simulink model "ES101A_DiagcMgr"  (R2013b)
settings: Solver=ode45  StartTime=0.0  StopTime=0.44  RelTol=1e-3
values from neighbouring files (symbols this model uses):
  BrdgVltg = DataDict.IpSignal    [ES101A_DiagcMgr_DataDict.m]
  DEM_CLEAR_PENDING = DataDict.Constant    [ES101A_DiagcMgr_DataDict.m]
  DEM_DTC_GROUP_ALL_DTCS = DataDict.Constant    [ES101A_DiagcMgr_DataDict.m]
  DFTAGICNTR_CNT_U08 = DataDict.Constant    [ES101A_DiagcMgr_DataDict.m]
  DIAGCMGR_NTCINFOSTSTESTFAILD_CNT_U08 = DataDict.Constant    [ES101A_DiagcMgr_DataDict.m]
  DIAGCMGR_NTCINFOSTSTESTFAILDTHISIGNCYC_CNT_U08 = DataDict.Constant    [ES101A_DiagcMgr_DataDict.m]
  DIAGCMGR_NTCINFOSTSTESTNOTCMPLTHISIGNCYC_CNT_U08 = DataDict.Constant    [ES101A_DiagcMgr_DataDict.m]
  DiagcMgrFltResp = DataDict.Calibration    [ES101A_DiagcMgr_DataDict.m]
  DiagcMgrNtcFltAry = DataDict.NVM    [ES101A_DiagcMgr_DataDict.m]
  DIAGCSTSCTRLDSHTDWNFLTPRSNT_CNT_U16 = DataDict.Constant    [ES101A_DiagcMgr_DataDict.m]
  DIAGCSTSDFTHWAG_CNT_U16 = DataDict.Constant    [ES101A_DiagcMgr_DataDict.m]
  DIAGCSTSDFTHWAGSERLCOMEXPRTVAL_CNT_U16 = DataDict.Constant    [ES101A_DiagcMgr_DataDict.m]
  DIAGCSTSDFTVEHSPD_CNT_U16 = DataDict.Constant    [ES101A_DiagcMgr_DataDict.m]
  DIAGCSTSININVAL_CNT_U16 = DataDict.Constant    [ES101A_DiagcMgr_DataDict.m]
  DIAGCSTSIVTR1INACTV_CNT_U16 = DataDict.Constant    [ES101A_DiagcMgr_DataDict.m]
  DIAGCSTSIVTR2INACTV_CNT_U16 = DataDict.Constant    [ES101A_DiagcMgr_DataDict.m]
  DIAGCSTSLIMDTPRFMNC_CNT_U16 = DataDict.Constant    [ES101A_DiagcMgr_DataDict.m]
  DIAGCSTSRAMPTOZEROFLTPRSNT_CNT_U16 = DataDict.Constant    [ES101A_DiagcMgr_DataDict.m]
  DIAGCSTSWHLIMBREJCTNDI_CNT_U16 = DataDict.Constant    [ES101A_DiagcMgr_DataDict.m]
  DTCIDXSTSFAIL_CNT_U08 = DataDict.Constant    [ES101A_DiagcMgr_DataDict.m]
  DTCIDXSTSNONTC_CNT_U08 = DataDict.Constant    [ES101A_DiagcMgr_DataDict.m]
  DTCIDXSTSNORES_CNT_U08 = DataDict.Constant    [ES101A_DiagcMgr_DataDict.m]
  DTCIDXSTSPASS_CNT_U08 = DataDict.Constant    [ES101A_DiagcMgr_DataDict.m]
  DTCIDXSTSUPDCFMD_CNT_U08 = DataDict.Constant    [ES101A_DiagcMgr_DataDict.m]
  ELECGLBPRM_IVTRCNT_CNT_U08 = DataDict.ConfigParam    [ES101A_DiagcMgr_DataDict.m]
  FLTINJ_DIAGCMGR_DIAGCSTSIVTR1INACTV = DataDict.Constant    [ES101A_DiagcMgr_DataDict.m]
  FLTINJ_DIAGCMGR_DIAGCSTSIVTR2INACTV = DataDict.Constant    [ES101A_DiagcMgr_DataDict.m]
  HwTq = DataDict.IpSignal    [ES101A_DiagcMgr_DataDict.m]
  IgnCntr = DataDict.IpSignal    [ES101A_DiagcMgr_DataDict.m]
  MAXDEBCNTRVAL_CNT_S16 = DataDict.Constant    [ES101A_DiagcMgr_DataDict.m]
  MAXRAMPRATE_ULSPERSEC_F32 = DataDict.Constant    [ES101A_DiagcMgr_DataDict.m]
  MINDEBCNTRVAL_CNT_S16 = DataDict.Constant    [ES101A_DiagcMgr_DataDict.m]
  MINRAMPRATE_ULSPERSEC_F32 = DataDict.Constant    [ES101A_DiagcMgr_DataDict.m]
  SCAMOTTQCMDTOONE_ULS_F32 = DataDict.Constant    [ES101A_DiagcMgr_DataDict.m]
  SCAMOTTQCMDTOZERO_ULS_F32 = DataDict.Constant    [ES101A_DiagcMgr_DataDict.m]
  SysSt = DataDict.IpSignal    [ES101A_DiagcMgr_DataDict.m]
  VehSpd = DataDict.IpSignal    [ES101A_DiagcMgr_DataDict.m]
undefined symbols (not defined in the file or in its folder): ActvMotTqCmdSca, ActvRampRate, AgiCntr, Dem_DTCFormatType, Dem_DTCOriginType, Dem_EventStatusType, DiagcData, DiagcMgrNtcMap, DiagcSts, DtcEnaMask, EcuT, HistNtcFltAry, MicroDiagcData, MotTq, NtcNr, NtcNrWithResd1, NtcStInfo, ProxySetNtcData, Sts, SysSt1, TOTNROFDTC_CNT_U08
libraries: simulink x151, FloatToFixd x5, NxtrNvM x4
(part 13 of 13)

== system ES101A_DiagcMgr/DiagcMgr/SetNtcStsCore/NtcNr is Valid/Diagnostics Not Inhibited/NtcEnabled/NTCSTS_PREFAILD/Update NtcInfoSts, DebCntr and Process RampRate/DebCntr = MAXDEBCNTRVAL_CNT_S16/ProcessRampResponse and DiagcSts/RapidShutdown Fault/Atomic Section2/Update Scale2 ==
  Action Port : ActionPort
  CopyRight2 : Subsystem  Description=|  mask(Copyright Information){none=on}
      | Copyright info block.                                               
      |                                                                     
      | Place copyright information at the top of every subsystem in design.
      mask prompts: none "No parameters"
      mask help: Place copyright information at the top of every subsystem in design.
      mask Display:
      | NxtrConf = 'Nexteer Confidential';
      | 
      | sys = bdroot; %handle for the current model ("system")
      | first = get_param(sys,'Created');
      | first = first(end-3:end);  %year is last four digits
      | 
      | last = get_param(sys,'LastModifiedDate');
      | if isempty(last)
      |     last = datestr(now,'yyyy');
      | else
      |     last = last(end-3:end);
      | end
      | 
      | if strcmp(first,last)
      |     fprintf('%s -- Copyright %s Nexteer',NxtrConf,first)
      | else
      |     fprintf('%s -- %s%s- %s Nexteer',NxtrConf,char(169),first,last)
      | end
  Scale Motor Torque Command to Zero : Constant  Value=SCAMOTTQCMDTOZERO_ULS_F32  OutDataTypeStr=single
  DiagcMgrActvMotTqCmdSca : Outport
  wires:
  Scale Motor Torque Command to Zero/1 -> DiagcMgrActvMotTqCmdSca/1

== system ES101A_DiagcMgr/DiagcMgr/SetNtcStsCore/NtcNr is Valid/Diagnostics Not Inhibited/NtcEnabled/NTCSTS_PREFAILD/Update NtcInfoSts, DebCntr and Process RampRate/DebCntr = MAXDEBCNTRVAL_CNT_S16/ProcessRampResponse and DiagcSts/RapidShutdown Fault/Atomic Section2/Update Scale3 ==
  Action Port : ActionPort
  CopyRight2 : Subsystem  Description=|  mask(Copyright Information){none=on}
      | Copyright info block.                                               
      |                                                                     
      | Place copyright information at the top of every subsystem in design.
      mask prompts: none "No parameters"
      mask help: Place copyright information at the top of every subsystem in design.
      mask Display:
      | NxtrConf = 'Nexteer Confidential';
      | 
      | sys = bdroot; %handle for the current model ("system")
      | first = get_param(sys,'Created');
      | first = first(end-3:end);  %year is last four digits
      | 
      | last = get_param(sys,'LastModifiedDate');
      | if isempty(last)
      |     last = datestr(now,'yyyy');
      | else
      |     last = last(end-3:end);
      | end
      | 
      | if strcmp(first,last)
      |     fprintf('%s -- Copyright %s Nexteer',NxtrConf,first)
      | else
      |     fprintf('%s -- %s%s- %s Nexteer',NxtrConf,char(169),first,last)
      | end
  Scale Motor Torque Command to Zero : Constant  Value=SCAMOTTQCMDTOZERO_ULS_F32  OutDataTypeStr=single
  ProxySetNtcMotTqCmdSca : Outport
  wires:
  Scale Motor Torque Command to Zero/1 -> ProxySetNtcMotTqCmdSca/1

== system ES101A_DiagcMgr/DiagcMgr/SetNtcStsCore/NtcNr is Valid/Diagnostics Not Inhibited/NtcEnabled/NTCSTS_PREFAILD/Update NtcInfoSts, DebCntr and Process RampRate/DebCntr = MAXDEBCNTRVAL_CNT_S16/ProcessRampResponse and DiagcSts/TimedShutdown Fault/Atomic Section2/CopyRight2 ==

== system ES101A_DiagcMgr/DiagcMgr/SetNtcStsCore/NtcNr is Valid/Diagnostics Not Inhibited/NtcEnabled/NTCSTS_PREFAILD/Update NtcInfoSts, DebCntr and Process RampRate/DebCntr = MAXDEBCNTRVAL_CNT_S16/ProcessRampResponse and DiagcSts/TimedShutdown Fault/Atomic Section2/Update Ramp Rate ==
  RampRate : Inport
  Action Port : ActionPort
  CopyRight2 : Subsystem  Description=|  mask(Copyright Information){none=on}
      | Copyright info block.                                               
      |                                                                     
      | Place copyright information at the top of every subsystem in design.
      mask prompts: none "No parameters"
      mask help: Place copyright information at the top of every subsystem in design.
      mask Display:
      | NxtrConf = 'Nexteer Confidential';
      | 
      | sys = bdroot; %handle for the current model ("system")
      | first = get_param(sys,'Created');
      | first = first(end-3:end);  %year is last four digits
      | 
      | last = get_param(sys,'LastModifiedDate');
      | if isempty(last)
      |     last = datestr(now,'yyyy');
      | else
      |     last = last(end-3:end);
      | end
      | 
      | if strcmp(first,last)
      |     fprintf('%s -- Copyright %s Nexteer',NxtrConf,first)
      | else
      |     fprintf('%s -- %s%s- %s Nexteer',NxtrConf,char(169),first,last)
      | end
  DiagcMgrActvRampRate : Outport
  wires:
  RampRate/1 -> DiagcMgrActvRampRate/1

== system ES101A_DiagcMgr/DiagcMgr/SetNtcStsCore/NtcNr is Valid/Diagnostics Not Inhibited/NtcEnabled/NTCSTS_PREFAILD/Update NtcInfoSts, DebCntr and Process RampRate/DebCntr = MAXDEBCNTRVAL_CNT_S16/ProcessRampResponse and DiagcSts/TimedShutdown Fault/Atomic Section2/Update Ramp Rate1 ==
  RampRate : Inport
  Action Port : ActionPort
  CopyRight2 : Subsystem  Description=|  mask(Copyright Information){none=on}
      | Copyright info block.                                               
      |                                                                     
      | Place copyright information at the top of every subsystem in design.
      mask prompts: none "No parameters"
      mask help: Place copyright information at the top of every subsystem in design.
      mask Display:
      | NxtrConf = 'Nexteer Confidential';
      | 
      | sys = bdroot; %handle for the current model ("system")
      | first = get_param(sys,'Created');
      | first = first(end-3:end);  %year is last four digits
      | 
      | last = get_param(sys,'LastModifiedDate');
      | if isempty(last)
      |     last = datestr(now,'yyyy');
      | else
      |     last = last(end-3:end);
      | end
      | 
      | if strcmp(first,last)
      |     fprintf('%s -- Copyright %s Nexteer',NxtrConf,first)
      | else
      |     fprintf('%s -- %s%s- %s Nexteer',NxtrConf,char(169),first,last)
      | end
  ProxySetNtcActvRampRate : Outport
  wires:
  RampRate/1 -> ProxySetNtcActvRampRate/1

== system ES101A_DiagcMgr/DiagcMgr/SetNtcStsCore/NtcNr is Valid/Diagnostics Not Inhibited/NtcEnabled/NTCSTS_PREFAILD/Update NtcInfoSts, DebCntr and Process RampRate/DebCntr = MAXDEBCNTRVAL_CNT_S16/ProcessRampResponse and DiagcSts/TimedShutdown Fault/Atomic Section2/Update Scale2 ==
  Action Port : ActionPort
  CopyRight2 : Subsystem  Description=|  mask(Copyright Information){none=on}
      | Copyright info block.                                               
      |                                                                     
      | Place copyright information at the top of every subsystem in design.
      mask prompts: none "No parameters"
      mask help: Place copyright information at the top of every subsystem in design.
      mask Display:
      | NxtrConf = 'Nexteer Confidential';
      | 
      | sys = bdroot; %handle for the current model ("system")
      | first = get_param(sys,'Created');
      | first = first(end-3:end);  %year is last four digits
      | 
      | last = get_param(sys,'LastModifiedDate');
      | if isempty(last)
      |     last = datestr(now,'yyyy');
      | else
      |     last = last(end-3:end);
      | end
      | 
      | if strcmp(first,last)
      |     fprintf('%s -- Copyright %s Nexteer',NxtrConf,first)
      | else
      |     fprintf('%s -- %s%s- %s Nexteer',NxtrConf,char(169),first,last)
      | end
  Scale Motor Torque Command to Zero : Constant  Value=SCAMOTTQCMDTOZERO_ULS_F32  OutDataTypeStr=single
  DiagcMgrActvMotTqCmdSca : Outport
  wires:
  Scale Motor Torque Command to Zero/1 -> DiagcMgrActvMotTqCmdSca/1

== system ES101A_DiagcMgr/DiagcMgr/SetNtcStsCore/NtcNr is Valid/Diagnostics Not Inhibited/NtcEnabled/NTCSTS_PREFAILD/Update NtcInfoSts, DebCntr and Process RampRate/DebCntr = MAXDEBCNTRVAL_CNT_S16/ProcessRampResponse and DiagcSts/TimedShutdown Fault/Atomic Section2/Update Scale3 ==
  Action Port : ActionPort
  CopyRight2 : Subsystem  Description=|  mask(Copyright Information){none=on}
      | Copyright info block.                                               
      |                                                                     
      | Place copyright information at the top of every subsystem in design.
      mask prompts: none "No parameters"
      mask help: Place copyright information at the top of every subsystem in design.
      mask Display:
      | NxtrConf = 'Nexteer Confidential';
      | 
      | sys = bdroot; %handle for the current model ("system")
      | first = get_param(sys,'Created');
      | first = first(end-3:end);  %year is last four digits
      | 
      | last = get_param(sys,'LastModifiedDate');
      | if isempty(last)
      |     last = datestr(now,'yyyy');
      | else
      |     last = last(end-3:end);
      | end
      | 
      | if strcmp(first,last)
      |     fprintf('%s -- Copyright %s Nexteer',NxtrConf,first)
      | else
      |     fprintf('%s -- %s%s- %s Nexteer',NxtrConf,char(169),first,last)
      | end
  Scale Motor Torque Command to Zero : Constant  Value=SCAMOTTQCMDTOZERO_ULS_F32  OutDataTypeStr=single
  ProxySetNtcMotTqCmdSca : Outport
  wires:
  Scale Motor Torque Command to Zero/1 -> ProxySetNtcMotTqCmdSca/1

== system ES101A_DiagcMgr/DiagcMgr/DiagcMgrPer2/Normal Periodic Processing/For All DTCs/For Each DTC/Check If DTC Status has Changed/DTC Status Changed OR DTC Update NOT Confirmed/Update DTC Status/Dtc Status is Failed/Update 'DTC Index Update Confirmed' Bit/StdRtn is E_OK/Set Bit 7 (DTC Update Confirmed)/CopyRight2 ==

== system ES101A_DiagcMgr/DiagcMgr/DiagcMgrPer2/Normal Periodic Processing/For All DTCs/For Each DTC/Check If DTC Status has Changed/DTC Status Changed OR DTC Update NOT Confirmed/Update DTC Status/Dtc Status is Passed/Update 'DTC Index Update Confirmed' Bit/StdRtn is E_OK/Set Bit 7 (DTC Update Confirmed)/CopyRight2 ==

== system ES101A_DiagcMgr/DiagcMgr/SetNtcStsCore/NtcNr is Valid/Diagnostics Not Inhibited/NtcEnabled/NTCSTS_FAILD/Update ISO Bits, Parameter Byte and AgiCntr /Check to Update Snapshot Data/UpdSnpshtData/Snapshot Data Enabled/While /While NTC Matches or Run out of Index/CopyRight2 ==

== system ES101A_DiagcMgr/DiagcMgr/SetNtcStsCore/NtcNr is Valid/Diagnostics Not Inhibited/NtcEnabled/NTCSTS_FAILD/Update ISO Bits, Parameter Byte and AgiCntr /Check to Update Snapshot Data/UpdSnpshtData/Snapshot Data Enabled/While /While NTC Matches or Run out of Index/Increment Snapshot Data Array Index ==
  Action Port : ActionPort
  Add : Sum
  Constant1 : Constant
  CopyRight2 : Subsystem  Description=|  mask(Copyright Information){none=on}
      | Copyright info block.                                               
      |                                                                     
      | Place copyright information at the top of every subsystem in design.
      mask prompts: none "No parameters"
      mask help: Place copyright information at the top of every subsystem in design.
      mask Display:
      | NxtrConf = 'Nexteer Confidential';
      | 
      | sys = bdroot; %handle for the current model ("system")
      | first = get_param(sys,'Created');
      | first = first(end-3:end);  %year is last four digits
      | 
      | last = get_param(sys,'LastModifiedDate');
      | if isempty(last)
      |     last = datestr(now,'yyyy');
      | else
      |     last = last(end-3:end);
      | end
      | 
      | if strcmp(first,last)
      |     fprintf('%s -- Copyright %s Nexteer',NxtrConf,first)
      | else
      |     fprintf('%s -- %s%s- %s Nexteer',NxtrConf,char(169),first,last)
      | end
  Snapshot Data Array Index : DataStoreRead  DataStoreName=SnpshtDataAryIdx
  "Snapshot Data Array Index " : DataStoreWrite  DataStoreName=SnpshtDataAryIdx
  wires:
  Constant1/1 -> Add/2
  Add/1 -> "Snapshot Data Array Index "/1
  Snapshot Data Array Index/1 -> Add/1

== system ES101A_DiagcMgr/DiagcMgr/SetNtcStsCore/NtcNr is Valid/Diagnostics Not Inhibited/NtcEnabled/NTCSTS_FAILD/Update ISO Bits, Parameter Byte and AgiCntr /Check to Update Snapshot Data/UpdSnpshtData/Snapshot Data Enabled/While /While NTC Matches or Run out of Index/NtcNr = 0 or Matching NtcNr ==
  NtcStInfo : Inport
  SnapshotDataBus : Inport  Port=2
  NtcNr : Inport  Port=3
  Action Port : ActionPort
  Bus Selector2 : BusSelector  OutputSignals=IgnCntr
  Bus Selector4 : BusSelector  OutputSignals=IgnCntr
  Constant : Constant  Value=0
  CopyRight2 : Subsystem  Description=|  mask(Copyright Information){none=on}
      | Copyright info block.                                               
      |                                                                     
      | Place copyright information at the top of every subsystem in design.
      mask prompts: none "No parameters"
      mask help: Place copyright information at the top of every subsystem in design.
      mask Display:
      | NxtrConf = 'Nexteer Confidential';
      | 
      | sys = bdroot; %handle for the current model ("system")
      | first = get_param(sys,'Created');
      | first = first(end-3:end);  %year is last four digits
      | 
      | last = get_param(sys,'LastModifiedDate');
      | if isempty(last)
      |     last = datestr(now,'yyyy');
      | else
      |     last = last(end-3:end);
      | end
      | 
      | if strcmp(first,last)
      |     fprintf('%s -- Copyright %s Nexteer',NxtrConf,first)
      | else
      |     fprintf('%s -- %s%s- %s Nexteer',NxtrConf,char(169),first,last)
      | end
  Data Store Write : DataStoreWrite  DataStoreName=SnpshtDataAryIdxInvld
  If : If  IfExpression=u1 == 1  ShowElse=off
  Relational Operator : RelationalOperator  Operator=<  OutDataTypeStr=boolean
  Selector : Selector  IndexMode=Zero-based  InputPortWidth=3  IndexOptions=Starting index (port)  Indices=[1 3]  OutputSizes=1
  Snapshot Data Array : DataStoreRead  DataStoreName=SnpshtDataAry
  Snapshot Data Array Index : DataStoreRead  DataStoreName=SnpshtDataAryIdx
  Snpsht Ign Cntr < Current IgnCntr : Subsystem
  wires:
  Constant/1 -> Data Store Write/1
  Bus Selector2/1 -> Relational Operator/2  "<IgnCntr>"
  SnapshotDataBus/1 -> Snpsht Ign Cntr < Current IgnCntr/2(SnapshotDataBus), Bus Selector2/1
  Selector/1 -> Bus Selector4/1
  Snapshot Data Array Index/1 -> Selector/2
  Snapshot Data Array/1 -> Selector/1
  Bus Selector4/1 -> Relational Operator/1  "<IgnCntr>"
  NtcStInfo/1 -> Snpsht Ign Cntr < Current IgnCntr/1(NtcStInfo)
  NtcNr/1 -> Snpsht Ign Cntr < Current IgnCntr/3(NtcNr)
  If/1 -> Snpsht Ign Cntr < Current IgnCntr/Action
  Relational Operator/1 -> If/1

== system ES101A_DiagcMgr/DiagcMgr/SetNtcStsCore/NtcNr is Valid/Diagnostics Not Inhibited/NtcEnabled/NTCSTS_PREFAILD/Update NtcInfoSts, DebCntr and Process RampRate/DebCntr = MAXDEBCNTRVAL_CNT_S16/Check to Update Snapshot Data/UpdSnpshtData/Snapshot Data Enabled/Initialize/CopyRight2 ==

== system ES101A_DiagcMgr/DiagcMgr/SetNtcStsCore/NtcNr is Valid/Diagnostics Not Inhibited/NtcEnabled/NTCSTS_PREFAILD/Update NtcInfoSts, DebCntr and Process RampRate/DebCntr = MAXDEBCNTRVAL_CNT_S16/Check to Update Snapshot Data/UpdSnpshtData/Snapshot Data Enabled/While /CopyRight2 ==

== system ES101A_DiagcMgr/DiagcMgr/SetNtcStsCore/NtcNr is Valid/Diagnostics Not Inhibited/NtcEnabled/NTCSTS_PREFAILD/Update NtcInfoSts, DebCntr and Process RampRate/DebCntr = MAXDEBCNTRVAL_CNT_S16/Check to Update Snapshot Data/UpdSnpshtData/Snapshot Data Enabled/While /While NTC Matches or Run out of Index ==
  IC : Inport
  cond : Inport  Port=2
  NtcNr : Inport  Port=3
  NtcStInfo : Inport  Port=4
  SnapshotDataBus : Inport  Port=5
  Bus Selector4 : BusSelector  OutputSignals=NtcNr
  CopyRight2 : Subsystem  Description=|  mask(Copyright Information){none=on}
      | Copyright info block.                                               
      |                                                                     
      | Place copyright information at the top of every subsystem in design.
      mask prompts: none "No parameters"
      mask help: Place copyright information at the top of every subsystem in design.
      mask Display:
      | NxtrConf = 'Nexteer Confidential';
      | 
      | sys = bdroot; %handle for the current model ("system")
      | first = get_param(sys,'Created');
      | first = first(end-3:end);  %year is last four digits
      | 
      | last = get_param(sys,'LastModifiedDate');
      | if isempty(last)
      |     last = datestr(now,'yyyy');
      | else
      |     last = last(end-3:end);
      | end
      | 
      | if strcmp(first,last)
      |     fprintf('%s -- Copyright %s Nexteer',NxtrConf,first)
      | else
      |     fprintf('%s -- %s%s- %s Nexteer',NxtrConf,char(169),first,last)
      | end
  Data Type Conversion : DataTypeConversion  OutDataTypeStr=uint16
  Data Type Conversion1 : DataTypeConversion  OutDataTypeStr=uint16
  If : If  NumInputs=2  IfExpression=u1 == 0|u2 == 1
  Increment Snapshot Data Array Index : Subsystem
  NtcNr = 0 or Matching NtcNr : Subsystem  TreatAsAtomicUnit=on
  Relational Operator1 : RelationalOperator  Operator===  OutDataTypeStr=boolean
  Selector : Selector  IndexMode=Zero-based  InputPortWidth=3  IndexOptions=Starting index (port)  Indices=[1 3]  OutputSizes=1
  Snapshot Data Array : DataStoreRead  DataStoreName=SnpshtDataAry
  Snapshot Data Array Index : DataStoreRead  DataStoreName=SnpshtDataAryIdx
  While Iterator : WhileIterator
  wires:
  Data Type Conversion/1 -> Relational Operator1/1, If/1
  Data Type Conversion1/1 -> Relational Operator1/2
  Relational Operator1/1 -> If/2
  NtcNr/1 -> Data Type Conversion1/1, NtcNr = 0 or Matching NtcNr/3(NtcNr)
  Bus Selector4/1 -> Data Type Conversion/1  "<NtcNr>"
  Selector/1 -> Bus Selector4/1
  Snapshot Data Array Index/1 -> Selector/2
  Snapshot Data Array/1 -> Selector/1
  If/2 -> Increment Snapshot Data Array Index/Action
  If/1 -> NtcNr = 0 or Matching NtcNr/Action
  cond/1 -> While Iterator/1
  IC/1 -> While Iterator/2
  SnapshotDataBus/1 -> NtcNr = 0 or Matching NtcNr/2(SnapshotDataBus)
  NtcStInfo/1 -> NtcNr = 0 or Matching NtcNr/1(NtcStInfo)

== system ES101A_DiagcMgr/DiagcMgr/SetNtcStsCore/NtcNr is Valid/Diagnostics Not Inhibited/NtcEnabled/NTCSTS_PREFAILD/Update NtcInfoSts, DebCntr and Process RampRate/DebCntr = MAXDEBCNTRVAL_CNT_S16/ProcessRampResponse and DiagcSts/ControlledShutdown Fault/Atomic Section2/Update Scale/CopyRight2 ==

== system ES101A_DiagcMgr/DiagcMgr/SetNtcStsCore/NtcNr is Valid/Diagnostics Not Inhibited/NtcEnabled/NTCSTS_PREFAILD/Update NtcInfoSts, DebCntr and Process RampRate/DebCntr = MAXDEBCNTRVAL_CNT_S16/ProcessRampResponse and DiagcSts/ControlledShutdown Fault/Atomic Section2/Update Scale1/CopyRight2 ==

== system ES101A_DiagcMgr/DiagcMgr/SetNtcStsCore/NtcNr is Valid/Diagnostics Not Inhibited/NtcEnabled/NTCSTS_PREFAILD/Update NtcInfoSts, DebCntr and Process RampRate/DebCntr = MAXDEBCNTRVAL_CNT_S16/ProcessRampResponse and DiagcSts/RapidShutdown Fault/Atomic Section2/Update Ramp Rate/CopyRight2 ==

== system ES101A_DiagcMgr/DiagcMgr/SetNtcStsCore/NtcNr is Valid/Diagnostics Not Inhibited/NtcEnabled/NTCSTS_PREFAILD/Update NtcInfoSts, DebCntr and Process RampRate/DebCntr = MAXDEBCNTRVAL_CNT_S16/ProcessRampResponse and DiagcSts/RapidShutdown Fault/Atomic Section2/Update Ramp Rate1/CopyRight2 ==

== system ES101A_DiagcMgr/DiagcMgr/SetNtcStsCore/NtcNr is Valid/Diagnostics Not Inhibited/NtcEnabled/NTCSTS_PREFAILD/Update NtcInfoSts, DebCntr and Process RampRate/DebCntr = MAXDEBCNTRVAL_CNT_S16/ProcessRampResponse and DiagcSts/RapidShutdown Fault/Atomic Section2/Update Scale2/CopyRight2 ==

== system ES101A_DiagcMgr/DiagcMgr/SetNtcStsCore/NtcNr is Valid/Diagnostics Not Inhibited/NtcEnabled/NTCSTS_PREFAILD/Update NtcInfoSts, DebCntr and Process RampRate/DebCntr = MAXDEBCNTRVAL_CNT_S16/ProcessRampResponse and DiagcSts/RapidShutdown Fault/Atomic Section2/Update Scale3/CopyRight2 ==

== system ES101A_DiagcMgr/DiagcMgr/SetNtcStsCore/NtcNr is Valid/Diagnostics Not Inhibited/NtcEnabled/NTCSTS_PREFAILD/Update NtcInfoSts, DebCntr and Process RampRate/DebCntr = MAXDEBCNTRVAL_CNT_S16/ProcessRampResponse and DiagcSts/TimedShutdown Fault/Atomic Section2/Update Ramp Rate/CopyRight2 ==

== system ES101A_DiagcMgr/DiagcMgr/SetNtcStsCore/NtcNr is Valid/Diagnostics Not Inhibited/NtcEnabled/NTCSTS_PREFAILD/Update NtcInfoSts, DebCntr and Process RampRate/DebCntr = MAXDEBCNTRVAL_CNT_S16/ProcessRampResponse and DiagcSts/TimedShutdown Fault/Atomic Section2/Update Ramp Rate1/CopyRight2 ==

== system ES101A_DiagcMgr/DiagcMgr/SetNtcStsCore/NtcNr is Valid/Diagnostics Not Inhibited/NtcEnabled/NTCSTS_PREFAILD/Update NtcInfoSts, DebCntr and Process RampRate/DebCntr = MAXDEBCNTRVAL_CNT_S16/ProcessRampResponse and DiagcSts/TimedShutdown Fault/Atomic Section2/Update Scale2/CopyRight2 ==

== system ES101A_DiagcMgr/DiagcMgr/SetNtcStsCore/NtcNr is Valid/Diagnostics Not Inhibited/NtcEnabled/NTCSTS_PREFAILD/Update NtcInfoSts, DebCntr and Process RampRate/DebCntr = MAXDEBCNTRVAL_CNT_S16/ProcessRampResponse and DiagcSts/TimedShutdown Fault/Atomic Section2/Update Scale3/CopyRight2 ==

== system ES101A_DiagcMgr/DiagcMgr/SetNtcStsCore/NtcNr is Valid/Diagnostics Not Inhibited/NtcEnabled/NTCSTS_FAILD/Update ISO Bits, Parameter Byte and AgiCntr /Check to Update Snapshot Data/UpdSnpshtData/Snapshot Data Enabled/While /While NTC Matches or Run out of Index/Increment Snapshot Data Array Index/CopyRight2 ==

== system ES101A_DiagcMgr/DiagcMgr/SetNtcStsCore/NtcNr is Valid/Diagnostics Not Inhibited/NtcEnabled/NTCSTS_FAILD/Update ISO Bits, Parameter Byte and AgiCntr /Check to Update Snapshot Data/UpdSnpshtData/Snapshot Data Enabled/While /While NTC Matches or Run out of Index/NtcNr = 0 or Matching NtcNr/CopyRight2 ==

== system ES101A_DiagcMgr/DiagcMgr/SetNtcStsCore/NtcNr is Valid/Diagnostics Not Inhibited/NtcEnabled/NTCSTS_FAILD/Update ISO Bits, Parameter Byte and AgiCntr /Check to Update Snapshot Data/UpdSnpshtData/Snapshot Data Enabled/While /While NTC Matches or Run out of Index/NtcNr = 0 or Matching NtcNr/Snpsht Ign Cntr < Current IgnCntr ==
  NtcStInfo : Inport
  SnapshotDataBus : Inport  Port=2
  NtcNr : Inport  Port=3
  Action Port : ActionPort  ActionType=then
  Bus Selector1 : BusSelector  OutputSignals=IgnCntr,MicroDiagcData,HwTq,MotTq,BrdgVltg,EcuT,SysSt,VehSpd
  CopyRight2 : Subsystem  Description=|  mask(Copyright Information){none=on}
      | Copyright info block.                                               
      |                                                                     
      | Place copyright information at the top of every subsystem in design.
      mask prompts: none "No parameters"
      mask help: Place copyright information at the top of every subsystem in design.
      mask Display:
      | NxtrConf = 'Nexteer Confidential';
      | 
      | sys = bdroot; %handle for the current model ("system")
      | first = get_param(sys,'Created');
      | first = first(end-3:end);  %year is last four digits
      | 
      | last = get_param(sys,'LastModifiedDate');
      | if isempty(last)
      |     last = datestr(now,'yyyy');
      | else
      |     last = last(end-3:end);
      | end
      | 
      | if strcmp(first,last)
      |     fprintf('%s -- Copyright %s Nexteer',NxtrConf,first)
      | else
      |     fprintf('%s -- %s%s- %s Nexteer',NxtrConf,char(169),first,last)
      | end
  Update Snapshot Data : Subsystem
  wires:
  SnapshotDataBus/1 -> Bus Selector1/1
  Bus Selector1/1 -> Update Snapshot Data/1(IgnCntr)  "<IgnCntr>"
  Bus Selector1/2 -> Update Snapshot Data/3(MicroDiagcData)  "<MicroDiagcData>"
  Bus Selector1/3 -> Update Snapshot Data/4(HwTq)  "<HwTq>"
  Bus Selector1/4 -> Update Snapshot Data/5(MotTq)  "<MotTq>"
  Bus Selector1/5 -> Update Snapshot Data/6(BrdgVltg)  "<BrdgVltg>"
  Bus Selector1/6 -> Update Snapshot Data/7(EcuT)  "<EcuT>"
  Bus Selector1/7 -> Update Snapshot Data/9(SysSt)  "<SysSt>"
  Bus Selector1/8 -> Update Snapshot Data/10(VehSpd)  "<VehSpd>"
  NtcStInfo/1 -> Update Snapshot Data/8(NtcStInfo)
  NtcNr/1 -> Update Snapshot Data/2(NtcNr)

== system ES101A_DiagcMgr/DiagcMgr/SetNtcStsCore/NtcNr is Valid/Diagnostics Not Inhibited/NtcEnabled/NTCSTS_PREFAILD/Update NtcInfoSts, DebCntr and Process RampRate/DebCntr = MAXDEBCNTRVAL_CNT_S16/Check to Update Snapshot Data/UpdSnpshtData/Snapshot Data Enabled/While /While NTC Matches or Run out of Index/CopyRight2 ==

== system ES101A_DiagcMgr/DiagcMgr/SetNtcStsCore/NtcNr is Valid/Diagnostics Not Inhibited/NtcEnabled/NTCSTS_PREFAILD/Update NtcInfoSts, DebCntr and Process RampRate/DebCntr = MAXDEBCNTRVAL_CNT_S16/Check to Update Snapshot Data/UpdSnpshtData/Snapshot Data Enabled/While /While NTC Matches or Run out of Index/Increment Snapshot Data Array Index ==
  Action Port : ActionPort
  Add : Sum
  Constant1 : Constant
  CopyRight2 : Subsystem  Description=|  mask(Copyright Information){none=on}
      | Copyright info block.                                               
      |                                                                     
      | Place copyright information at the top of every subsystem in design.
      mask prompts: none "No parameters"
      mask help: Place copyright information at the top of every subsystem in design.
      mask Display:
      | NxtrConf = 'Nexteer Confidential';
      | 
      | sys = bdroot; %handle for the current model ("system")
      | first = get_param(sys,'Created');
      | first = first(end-3:end);  %year is last four digits
      | 
      | last = get_param(sys,'LastModifiedDate');
      | if isempty(last)
      |     last = datestr(now,'yyyy');
      | else
      |     last = last(end-3:end);
      | end
      | 
      | if strcmp(first,last)
      |     fprintf('%s -- Copyright %s Nexteer',NxtrConf,first)
      | else
      |     fprintf('%s -- %s%s- %s Nexteer',NxtrConf,char(169),first,last)
      | end
  Snapshot Data Array Index : DataStoreRead  DataStoreName=SnpshtDataAryIdx
  "Snapshot Data Array Index " : DataStoreWrite  DataStoreName=SnpshtDataAryIdx
  wires:
  Constant1/1 -> Add/2
  Add/1 -> "Snapshot Data Array Index "/1
  Snapshot Data Array Index/1 -> Add/1

== system ES101A_DiagcMgr/DiagcMgr/SetNtcStsCore/NtcNr is Valid/Diagnostics Not Inhibited/NtcEnabled/NTCSTS_PREFAILD/Update NtcInfoSts, DebCntr and Process RampRate/DebCntr = MAXDEBCNTRVAL_CNT_S16/Check to Update Snapshot Data/UpdSnpshtData/Snapshot Data Enabled/While /While NTC Matches or Run out of Index/NtcNr = 0 or Matching NtcNr ==
  NtcStInfo : Inport
  SnapshotDataBus : Inport  Port=2
  NtcNr : Inport  Port=3
  Action Port : ActionPort
  Bus Selector2 : BusSelector  OutputSignals=IgnCntr
  Bus Selector4 : BusSelector  OutputSignals=IgnCntr
  Constant : Constant  Value=0
  CopyRight2 : Subsystem  Description=|  mask(Copyright Information){none=on}
      | Copyright info block.                                               
      |                                                                     
      | Place copyright information at the top of every subsystem in design.
      mask prompts: none "No parameters"
      mask help: Place copyright information at the top of every subsystem in design.
      mask Display:
      | NxtrConf = 'Nexteer Confidential';
      | 
      | sys = bdroot; %handle for the current model ("system")
      | first = get_param(sys,'Created');
      | first = first(end-3:end);  %year is last four digits
      | 
      | last = get_param(sys,'LastModifiedDate');
      | if isempty(last)
      |     last = datestr(now,'yyyy');
      | else
      |     last = last(end-3:end);
      | end
      | 
      | if strcmp(first,last)
      |     fprintf('%s -- Copyright %s Nexteer',NxtrConf,first)
      | else
      |     fprintf('%s -- %s%s- %s Nexteer',NxtrConf,char(169),first,last)
      | end
  Data Store Write : DataStoreWrite  DataStoreName=SnpshtDataAryIdxInvld
  If : If  IfExpression=u1 == 1  ShowElse=off
  Relational Operator : RelationalOperator  Operator=<  OutDataTypeStr=boolean
  Selector : Selector  IndexMode=Zero-based  InputPortWidth=3  IndexOptions=Starting index (port)  Indices=[1 3]  OutputSizes=1
  Snapshot Data Array : DataStoreRead  DataStoreName=SnpshtDataAry
  Snapshot Data Array Index : DataStoreRead  DataStoreName=SnpshtDataAryIdx
  Snpsht Ign Cntr < Current IgnCntr : Subsystem
  wires:
  Constant/1 -> Data Store Write/1
  Bus Selector2/1 -> Relational Operator/2  "<IgnCntr>"
  SnapshotDataBus/1 -> Snpsht Ign Cntr < Current IgnCntr/2(SnapshotDataBus), Bus Selector2/1
  Selector/1 -> Bus Selector4/1
  Snapshot Data Array Index/1 -> Selector/2
  Snapshot Data Array/1 -> Selector/1
  Bus Selector4/1 -> Relational Operator/1  "<IgnCntr>"
  NtcStInfo/1 -> Snpsht Ign Cntr < Current IgnCntr/1(NtcStInfo)
  NtcNr/1 -> Snpsht Ign Cntr < Current IgnCntr/3(NtcNr)
  If/1 -> Snpsht Ign Cntr < Current IgnCntr/Action
  Relational Operator/1 -> If/1

== system ES101A_DiagcMgr/DiagcMgr/SetNtcStsCore/NtcNr is Valid/Diagnostics Not Inhibited/NtcEnabled/NTCSTS_FAILD/Update ISO Bits, Parameter Byte and AgiCntr /Check to Update Snapshot Data/UpdSnpshtData/Snapshot Data Enabled/While /While NTC Matches or Run out of Index/NtcNr = 0 or Matching NtcNr/Snpsht Ign Cntr < Current IgnCntr/CopyRight2 ==

== system ES101A_DiagcMgr/DiagcMgr/SetNtcStsCore/NtcNr is Valid/Diagnostics Not Inhibited/NtcEnabled/NTCSTS_FAILD/Update ISO Bits, Parameter Byte and AgiCntr /Check to Update Snapshot Data/UpdSnpshtData/Snapshot Data Enabled/While /While NTC Matches or Run out of Index/NtcNr = 0 or Matching NtcNr/Snpsht Ign Cntr < Current IgnCntr/Update Snapshot Data ==
  IgnCntr : Inport
  NtcNr : Inport  Port=2
  MicroDiagcData : Inport  Port=3
  HwTq : Inport  Port=4
  MotTq : Inport  Port=5
  BrdgVltg : Inport  Port=6
  EcuT : Inport  Port=7
  NtcStInfo : Inport  Port=8
  SysSt : Inport  Port=9
  VehSpd : Inport  Port=10
  Assignment1 : Assignment  IndexMode=Zero-based  IndexOptions=Index vector (port)  Indices=1  OutputSizes=1
  Bus Assignment3 : BusAssignment  AssignedSignals=MicroDiagcData,HwTq,MotTq,IgnCntr,BrdgVltg,EcuT,NtcNr,NtcStInfo,SysSt,VehSpd
  Constant : Constant  OutDataTypeStr=uint8
  CopyRight2 : Subsystem  Description=|  mask(Copyright Information){none=on}
      | Copyright info block.                                               
      |                                                                     
      | Place copyright information at the top of every subsystem in design.
      mask prompts: none "No parameters"
      mask help: Place copyright information at the top of every subsystem in design.
      mask Display:
      | NxtrConf = 'Nexteer Confidential';
      | 
      | sys = bdroot; %handle for the current model ("system")
      | first = get_param(sys,'Created');
      | first = first(end-3:end);  %year is last four digits
      | 
      | last = get_param(sys,'LastModifiedDate');
      | if isempty(last)
      |     last = datestr(now,'yyyy');
      | else
      |     last = last(end-3:end);
      | end
      | 
      | if strcmp(first,last)
      |     fprintf('%s -- Copyright %s Nexteer',NxtrConf,first)
      | else
      |     fprintf('%s -- %s%s- %s Nexteer',NxtrConf,char(169),first,last)
      | end
  Data Store Write : DataStoreWrite  DataStoreName=SnpshtDataAry
  Data Type Conversion : DataTypeConversion  OutDataTypeStr=Enum: NtcNrWithResd1
  Set Ram Block Status : NxtrNvM/Set Ram Block Status  FuncName=Set Ram Block Status  NvMBlockName=SnpShtDataAry  VoidFuncRtn=on  BlockChanged_DSN=NvMSRBS_BlockChanged  Return_DSN=NvMSRBS_Return
      settings: AttributesFormatString=%<FuncName>
  Snapshot Data Array : DataStoreRead  DataStoreName=SnpshtDataAry
  Snapshot Data Array Index : DataStoreRead  DataStoreName=SnpshtDataAryIdx
  wires:
  Constant/1 -> Set Ram Block Status/1
  Assignment1/1 -> Data Store Write/1
  Snapshot Data Array Index/1 -> Assignment1/3
  Snapshot Data Array/1 -> Bus Assignment3/1, Assignment1/1
  Bus Assignment3/1 -> Assignment1/2
  MicroDiagcData/1 -> Bus Assignment3/2
  HwTq/1 -> Bus Assignment3/3
  MotTq/1 -> Bus Assignment3/4
  IgnCntr/1 -> Bus Assignment3/5
  BrdgVltg/1 -> Bus Assignment3/6
  EcuT/1 -> Bus Assignment3/7
  NtcNr/1 -> Data Type Conversion/1
  NtcStInfo/1 -> Bus Assignment3/9
  SysSt/1 -> Bus Assignment3/10
  VehSpd/1 -> Bus Assignment3/11
  Data Type Conversion/1 -> Bus Assignment3/8

== system ES101A_DiagcMgr/DiagcMgr/SetNtcStsCore/NtcNr is Valid/Diagnostics Not Inhibited/NtcEnabled/NTCSTS_PREFAILD/Update NtcInfoSts, DebCntr and Process RampRate/DebCntr = MAXDEBCNTRVAL_CNT_S16/Check to Update Snapshot Data/UpdSnpshtData/Snapshot Data Enabled/While /While NTC Matches or Run out of Index/Increment Snapshot Data Array Index/CopyRight2 ==

== system ES101A_DiagcMgr/DiagcMgr/SetNtcStsCore/NtcNr is Valid/Diagnostics Not Inhibited/NtcEnabled/NTCSTS_PREFAILD/Update NtcInfoSts, DebCntr and Process RampRate/DebCntr = MAXDEBCNTRVAL_CNT_S16/Check to Update Snapshot Data/UpdSnpshtData/Snapshot Data Enabled/While /While NTC Matches or Run out of Index/NtcNr = 0 or Matching NtcNr/CopyRight2 ==

== system ES101A_DiagcMgr/DiagcMgr/SetNtcStsCore/NtcNr is Valid/Diagnostics Not Inhibited/NtcEnabled/NTCSTS_PREFAILD/Update NtcInfoSts, DebCntr and Process RampRate/DebCntr = MAXDEBCNTRVAL_CNT_S16/Check to Update Snapshot Data/UpdSnpshtData/Snapshot Data Enabled/While /While NTC Matches or Run out of Index/NtcNr = 0 or Matching NtcNr/Snpsht Ign Cntr < Current IgnCntr ==
  NtcStInfo : Inport
  SnapshotDataBus : Inport  Port=2
  NtcNr : Inport  Port=3
  Action Port : ActionPort
  Bus Selector1 : BusSelector  OutputSignals=IgnCntr,MicroDiagcData,HwTq,MotTq,BrdgVltg,EcuT,SysSt,VehSpd
  CopyRight2 : Subsystem  Description=|  mask(Copyright Information){none=on}
      | Copyright info block.                                               
      |                                                                     
      | Place copyright information at the top of every subsystem in design.
      mask prompts: none "No parameters"
      mask help: Place copyright information at the top of every subsystem in design.
      mask Display:
      | NxtrConf = 'Nexteer Confidential';
      | 
      | sys = bdroot; %handle for the current model ("system")
      | first = get_param(sys,'Created');
      | first = first(end-3:end);  %year is last four digits
      | 
      | last = get_param(sys,'LastModifiedDate');
      | if isempty(last)
      |     last = datestr(now,'yyyy');
      | else
      |     last = last(end-3:end);
      | end
      | 
      | if strcmp(first,last)
      |     fprintf('%s -- Copyright %s Nexteer',NxtrConf,first)
      | else
      |     fprintf('%s -- %s%s- %s Nexteer',NxtrConf,char(169),first,last)
      | end
  Update Snapshot Data : Subsystem
  wires:
  SnapshotDataBus/1 -> Bus Selector1/1
  Bus Selector1/1 -> Update Snapshot Data/1(IgnCntr)  "<IgnCntr>"
  Bus Selector1/2 -> Update Snapshot Data/3(MicroDiagcData)  "<MicroDiagcData>"
  Bus Selector1/3 -> Update Snapshot Data/4(HwTq)  "<HwTq>"
  Bus Selector1/4 -> Update Snapshot Data/5(MotTq)  "<MotTq>"
  Bus Selector1/5 -> Update Snapshot Data/6(BrdgVltg)  "<BrdgVltg>"
  Bus Selector1/6 -> Update Snapshot Data/7(EcuT)  "<EcuT>"
  Bus Selector1/7 -> Update Snapshot Data/9(SysSt)  "<SysSt>"
  Bus Selector1/8 -> Update Snapshot Data/10(VehSpd)  "<VehSpd>"
  NtcStInfo/1 -> Update Snapshot Data/8(NtcStInfo)
  NtcNr/1 -> Update Snapshot Data/2(NtcNr)

== system ES101A_DiagcMgr/DiagcMgr/SetNtcStsCore/NtcNr is Valid/Diagnostics Not Inhibited/NtcEnabled/NTCSTS_FAILD/Update ISO Bits, Parameter Byte and AgiCntr /Check to Update Snapshot Data/UpdSnpshtData/Snapshot Data Enabled/While /While NTC Matches or Run out of Index/NtcNr = 0 or Matching NtcNr/Snpsht Ign Cntr < Current IgnCntr/Update Snapshot Data/CopyRight2 ==

== system ES101A_DiagcMgr/DiagcMgr/SetNtcStsCore/NtcNr is Valid/Diagnostics Not Inhibited/NtcEnabled/NTCSTS_PREFAILD/Update NtcInfoSts, DebCntr and Process RampRate/DebCntr = MAXDEBCNTRVAL_CNT_S16/Check to Update Snapshot Data/UpdSnpshtData/Snapshot Data Enabled/While /While NTC Matches or Run out of Index/NtcNr = 0 or Matching NtcNr/Snpsht Ign Cntr < Current IgnCntr/CopyRight2 ==

== system ES101A_DiagcMgr/DiagcMgr/SetNtcStsCore/NtcNr is Valid/Diagnostics Not Inhibited/NtcEnabled/NTCSTS_PREFAILD/Update NtcInfoSts, DebCntr and Process RampRate/DebCntr = MAXDEBCNTRVAL_CNT_S16/Check to Update Snapshot Data/UpdSnpshtData/Snapshot Data Enabled/While /While NTC Matches or Run out of Index/NtcNr = 0 or Matching NtcNr/Snpsht Ign Cntr < Current IgnCntr/Update Snapshot Data ==
  IgnCntr : Inport
  NtcNr : Inport  Port=2
  MicroDiagcData : Inport  Port=3
  HwTq : Inport  Port=4
  MotTq : Inport  Port=5
  BrdgVltg : Inport  Port=6
  EcuT : Inport  Port=7
  NtcStInfo : Inport  Port=8
  SysSt : Inport  Port=9
  VehSpd : Inport  Port=10
  Assignment1 : Assignment  IndexMode=Zero-based  IndexOptions=Index vector (port)  Indices=1  OutputSizes=1
  Bus Assignment3 : BusAssignment  AssignedSignals=MicroDiagcData,HwTq,MotTq,IgnCntr,BrdgVltg,EcuT,NtcNr,NtcStInfo,SysSt,VehSpd
  Constant : Constant  OutDataTypeStr=uint8
  CopyRight2 : Subsystem  Description=|  mask(Copyright Information){none=on}
      | Copyright info block.                                               
      |                                                                     
      | Place copyright information at the top of every subsystem in design.
      mask prompts: none "No parameters"
      mask help: Place copyright information at the top of every subsystem in design.
      mask Display:
      | NxtrConf = 'Nexteer Confidential';
      | 
      | sys = bdroot; %handle for the current model ("system")
      | first = get_param(sys,'Created');
      | first = first(end-3:end);  %year is last four digits
      | 
      | last = get_param(sys,'LastModifiedDate');
      | if isempty(last)
      |     last = datestr(now,'yyyy');
      | else
      |     last = last(end-3:end);
      | end
      | 
      | if strcmp(first,last)
      |     fprintf('%s -- Copyright %s Nexteer',NxtrConf,first)
      | else
      |     fprintf('%s -- %s%s- %s Nexteer',NxtrConf,char(169),first,last)
      | end
  Data Store Write : DataStoreWrite  DataStoreName=SnpshtDataAry
  Data Type Conversion : DataTypeConversion  OutDataTypeStr=Enum: NtcNrWithResd1
  Set Ram Block Status : NxtrNvM/Set Ram Block Status  FuncName=Set Ram Block Status  NvMBlockName=SnpShtDataAry  VoidFuncRtn=on  BlockChanged_DSN=NvMSRBS_BlockChanged  Return_DSN=NvMSRBS_Return
      settings: AttributesFormatString=%<FuncName>
  Snapshot Data Array : DataStoreRead  DataStoreName=SnpshtDataAry
  Snapshot Data Array Index : DataStoreRead  DataStoreName=SnpshtDataAryIdx
  wires:
  Constant/1 -> Set Ram Block Status/1
  Assignment1/1 -> Data Store Write/1
  Snapshot Data Array Index/1 -> Assignment1/3
  Snapshot Data Array/1 -> Bus Assignment3/1, Assignment1/1
  Bus Assignment3/1 -> Assignment1/2
  MicroDiagcData/1 -> Bus Assignment3/2
  HwTq/1 -> Bus Assignment3/3
  MotTq/1 -> Bus Assignment3/4
  IgnCntr/1 -> Bus Assignment3/5
  BrdgVltg/1 -> Bus Assignment3/6
  EcuT/1 -> Bus Assignment3/7
  NtcNr/1 -> Data Type Conversion/1
  NtcStInfo/1 -> Bus Assignment3/9
  SysSt/1 -> Bus Assignment3/10
  VehSpd/1 -> Bus Assignment3/11
  Data Type Conversion/1 -> Bus Assignment3/8

== system ES101A_DiagcMgr/DiagcMgr/SetNtcStsCore/NtcNr is Valid/Diagnostics Not Inhibited/NtcEnabled/NTCSTS_PREFAILD/Update NtcInfoSts, DebCntr and Process RampRate/DebCntr = MAXDEBCNTRVAL_CNT_S16/Check to Update Snapshot Data/UpdSnpshtData/Snapshot Data Enabled/While /While NTC Matches or Run out of Index/NtcNr = 0 or Matching NtcNr/Snpsht Ign Cntr < Current IgnCntr/Update Snapshot Data/CopyRight2 ==
